simulink model "DriveCycle_e8_IPMSM_HWJandVent_ROM"  (R2021b)
settings: Solver=VariableStepAuto  StartTime=0.0  StopTime=2474  FixedStep=1e-2  RelTol=1e-3  AbsTol=1e-3
model workspace (MAT data in the model file):
  AdjacencyMat = [0 0 0 0 0 0 0 0 0 0 0 0 ... (15129 elements, 123x123)]
  CapMat = [1e+20 2196.70091586 387.653102799 193.8265514 1962.34710525 387.653102799 193.8265514 1962.34710525 1266.59353814 268.053957132 416.539515956 175.715078 ... (123 elements, 123x1)]
  CoolantArrayIdxs = [20 21 22 23 24 25 26 27 35 36 37 84 ... (19 elements, 19x1)]
  Friction_Loss_Mat = [0 0 0 0 0 0 0 0 0 0 0 0 ... (2340 elements, 39x60)]
  InletCoolIdxs = [37; 38]
  Iron_Loss_Rotor_Back_Iron_Mat = [0.0117705351991 0.0198175800092 0.0246057415963 0.0256631766661 0.0240576767285 0.0207771722396 0.0168311502834 0.0133395315761 0.0115512535049 0.0120779527774 0.0143067244388 0.0171516443454 ... (2340 elements, 39x60)]
  Iron_Loss_Rotor_Pole_Mat = [1.45649756865 1.4525095653 1.42942652973 1.39109338754 1.34251579982 1.287439524 1.22885659237 1.16930852698 1.11098912611 1.05484046499 0.999976047808 0.944563732162 ... (2340 elements, 39x60)]
  Iron_Loss_Rotor_Tooth_Mat = [0 0 0 0 0 0 0 0 0 0 0 0 ... (2340 elements, 39x60)]
  Iron_Loss_Stator_Back_Iron_Mat = [38.5419456951 37.774471759 36.7837540443 35.6885758764 34.5272571596 33.3324529178 32.136302555 30.9744032473 29.8863152048 28.8790573391 27.8876077961 26.8074662049 ... (2340 elements, 39x60)]
  Iron_Loss_Stator_Tooth_Mat = [42.0610884508 41.0604961882 40.1804594162 39.4285940164 38.704339026 37.9602455604 37.1844153901 36.3902226975 35.6050856075 34.8287218867 34.0007237809 33.0439458619 ... (2340 elements, 39x60)]
  LossDistrForEachType = [0 0 0 0 0 0 0 0 0 0 0 0 ... (1968 elements, 16x123)]
  Magnet_Loss_Mat = [0.0995193918038 0.0928899922278 0.0868628846748 0.0818830115456 0.0774722500184 0.0732395922727 0.0687988836096 0.0636930921801 0.0573503948699 0.0496000064543 0.0410757743485 0.0326817704515 ... (2340 elements, 39x60)]
  OutletCoolIdxs = [20; 107]
  ResMat = [0 2.49009256841 6.64572241429 1000000000 1.39790968864 6.64402802995 1000000000 1.39156082742 1000000000 1000000000 1000000000 1000000000 ... (15129 elements, 123x123)]
  RotorCopperTempCoefResistivity = 0.00393
  Rotor_Cage_Loss_Mat = [0 0 0 0 0 0 0 0 0 0 0 0 ... (2340 elements, 39x60)]
  ShaftTorqueVec = [-287.262157301 -272.268610731 -257.275064161 -242.281517591 -227.287971021 -212.294424451 -197.300877881 -182.307331311 -167.31378474 -152.32023817 -137.3266916 -122.33314503 ... (39 elements, 1x39)]
  Sig : Simulink.Signal (value not decoded)
  SpeedVec = [500 661.016949153 822.033898305 983.050847458 1144.06779661 1305.08474576 1466.10169492 1627.11864407 1788.13559322 1949.15254237 2110.16949153 2271.18644068 ... (60 elements, 1x60)]
  StateSpaceND : object (value not decoded)
  StatorCopperTempCoefResistivity = 0.00393
  Stator_Copper_Loss_Mat = [3925.33912093 3510.19452231 3089.33767218 2711.80000483 2370.99356953 2062.06508217 1781.35176729 1526.02799256 1293.87708125 1083.15658499 892.54525431 720.809889245 ... (2340 elements, 39x60)]
  Stray_Load_Loss_Mat = [0 0 0 0 0 0 0 0 0 0 0 0 ... (2340 elements, 39x60)]
  Stray_Loss_Stator_Iron_Proportion = 0.95
  Tgiven = 20
  TnodesInit = [25 25 25 25 25 25 25 25 25 25 25 25 ... (123 elements, 123x1)]
  TrefRotor = 20
  TrefStator = 20
  Windage_Loss_Mat = [0 0 0 0 0 0 0 0 0 0 0 0 ... (2340 elements, 39x60)]
libraries: mcadROM_lib x4, autolibshared x1, simulink x1
(part 2 of 2)

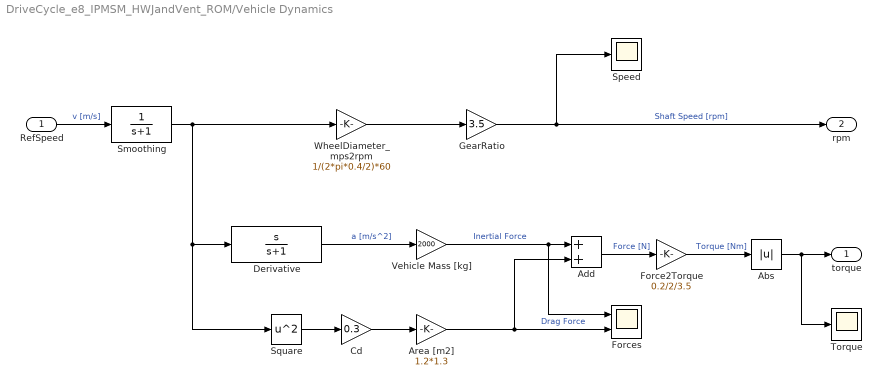
== system DriveCycle_e8_IPMSM_HWJandVent_ROM/Vehicle Dynamics ==
  RefSpeed : Inport
  Abs : Abs
  Add : Sum
  Area [m2] : Gain  Gain=1.2*1.3
  Cd : Gain  Gain=0.3
  Derivative : TransferFcn  Numerator=[1 0]  Denominator=[1, 1]
  Force2Torque : Gain  Gain=0.2/2/3.5
  Forces : Scope  NumInputPorts=2
  GearRatio : Gain  Gain=3.5
  Smoothing : TransferFcn  Denominator=[1 1]
  Speed : Scope
  Square : Math  Operator=square  SaturateOnIntegerOverflow=on
  Torque : Scope
  Vehicle Mass [kg] : Gain  Gain=2000
  WheelDiameter_mps2rpm : Gain  Gain=1/(2*pi*0.4/2)*60
  torque : Outport
  rpm : Outport  Port=2
  wires:
  GearRatio/1 -> Speed/1, rpm/1  "Shaft Speed [rpm]"
  WheelDiameter_mps2rpm/1 -> GearRatio/1
  Derivative/1 -> Vehicle Mass [kg]/1  "a [m/s^2]"
  Add/1 -> Force2Torque/1  "Force [N]"
  Vehicle Mass [kg]/1 -> Forces/1, Add/1  "Inertial Force"
  Area [m2]/1 -> Forces/2, Add/2  "Drag Force"
  Square/1 -> Cd/1
  Cd/1 -> Area [m2]/1
  RefSpeed/1 -> Smoothing/1  "v [m/s]"
  Smoothing/1 -> Derivative/1, Square/1, WheelDiameter_mps2rpm/1
  Force2Torque/1 -> Abs/1  "Torque [Nm]"
  Abs/1 -> Torque/1, torque/1

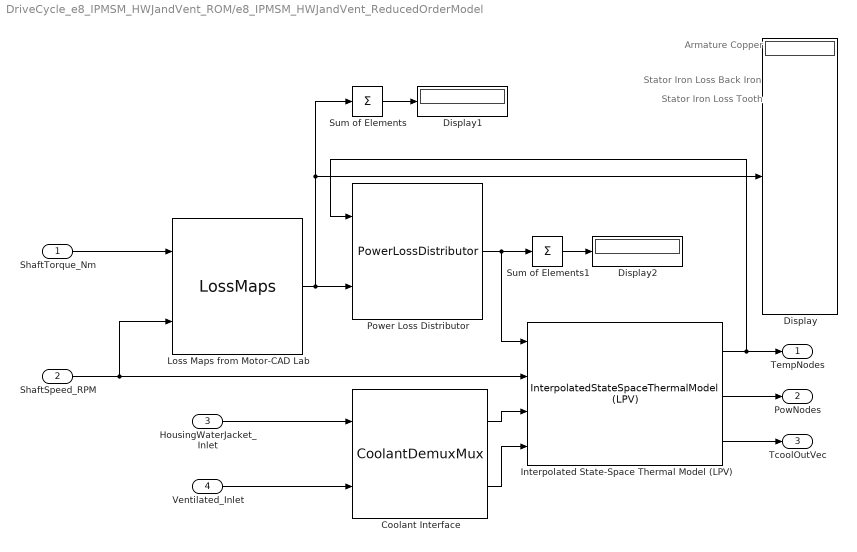
== system DriveCycle_e8_IPMSM_HWJandVent_ROM/e8_IPMSM_HWJandVent_ReducedOrderModel ==
  note: Stator Iron Loss Tooth
  note: Stator Iron Loss Back Iron
  note: Armature Copper
  ShaftTorque_Nm : Inport
  ShaftSpeed_RPM : Inport  Port=2
  HousingWaterJacket_Inlet : Inport  Port=3
  Ventilated_Inlet : Inport  Port=4
  Coolant Interface : mcadROM_lib/CoolantDemuxMux  numCoolSys=2
  Display : Display
  Display1 : Display
  Display2 : Display
  Interpolated State-Space Thermal Model (LPV) : mcadROM_lib/InterpolatedStateSpaceThermalModel (LPV)  StateSpaceND=StateSpaceND  CoolAdjMat=AdjacencyMat  CoolantArrayIdxs=CoolantArrayIdxs  InletCoolantIdxs=InletCoolIdxs  OutletCoolantIdxs=OutletCoolIdxs  TnodesInit=TnodesInit
  Loss Maps from Motor-CAD Lab : mcadROM_lib/LossMaps  ShaftTorqueVec=ShaftTorqueVec  SpeedVec=SpeedVec  Stator_Copper_Loss_Mat=Stator_Copper_Loss_Mat  Rotor_Cage_Loss_Mat=Rotor_Cage_Loss_Mat  Iron_Loss_Stator_Back_Iron_Mat=Iron_Loss_Stator_Back_Iron_Mat  Iron_Loss_Stator_Tooth_Mat=Iron_Loss_Stator_Tooth_Mat  Stray_Loss_Stator_Iron_Proportion=Stray_Loss_Stator_Iron_Proportion  Stray_Load_Loss_Mat=Stray_Load_Loss_Mat  Magnet_Loss_Mat=Magnet_Loss_Mat  Iron_Loss_Rotor_Pole_Mat=Iron_Loss_Rotor_Pole_Mat  Iron_Loss_Rotor_Back_Iron_Mat=Iron_Loss_Rotor_Back_Iron_Mat  Iron_Loss_Rotor_Tooth_Mat=Iron_Loss_Rotor_Tooth_Mat  Friction_Loss_Mat=Friction_Loss_Mat  Windage_Loss_Mat=Windage_Loss_Mat
  Power Loss Distributor : mcadROM_lib/PowerLossDistributor  TrefStator=20  StatorCopperTempCoefResistivity=StatorCopperTempCoefResistivity  TrefRotor=20  RotorCopperTempCoefResistivity=1e-5  LossDistrForEachType=LossDistrForEachType  CapMat=CapMat  CoolantArrayIdxs=CoolantArrayIdxs
  Sum of Elements : Sum  Inputs=+
  Sum of Elements1 : Sum  Inputs=+
  TempNodes : Outport
  PowNodes : Outport  Port=2
  TcoolOutVec : Outport  Port=3
  wires:
  Interpolated State-Space Thermal Model (LPV)/1 -> Power Loss Distributor/1, TempNodes/1
  HousingWaterJacket_Inlet/1 -> Coolant Interface/1
  Interpolated State-Space Thermal Model (LPV)/3 -> TcoolOutVec/1
  Loss Maps from Motor-CAD Lab/1 -> Power Loss Distributor/2, Sum of Elements/1, Display/1
  Coolant Interface/1 -> Interpolated State-Space Thermal Model (LPV)/3
  Ventilated_Inlet/1 -> Coolant Interface/2
  ShaftTorque_Nm/1 -> Loss Maps from Motor-CAD Lab/1
  Coolant Interface/2 -> Interpolated State-Space Thermal Model (LPV)/4
  Interpolated State-Space Thermal Model (LPV)/2 -> PowNodes/1
  ShaftSpeed_RPM/1 -> Interpolated State-Space Thermal Model (LPV)/2, Loss Maps from Motor-CAD Lab/2
  Sum of Elements/1 -> Display1/1
  Sum of Elements1/1 -> Display2/1
  Power Loss Distributor/1 -> Interpolated State-Space Thermal Model (LPV)/1, Sum of Elements1/1
